simulink model "HPTtest"  (R2025a)
settings: Solver=VariableStepAuto  StartTime=0.0  StopTime=10.0  RelTol=1e-3
undefined symbols (not defined in the file): Eff_hpt_map, effMod_HPT, norm_flow_hpt, norm_speed_hpt, Torque_hpt_map
settings Model: Creator=ramch  LastModifiedBy=ramch

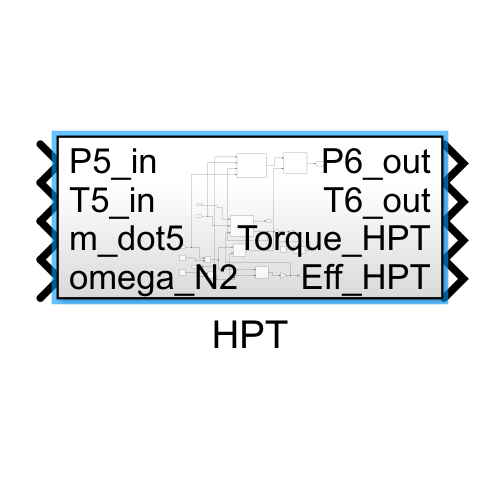
[thumbnail: Simulink's stored preview of the top-level diagram]
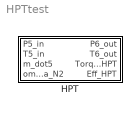
== system HPTtest ==
  HPT : Subsystem

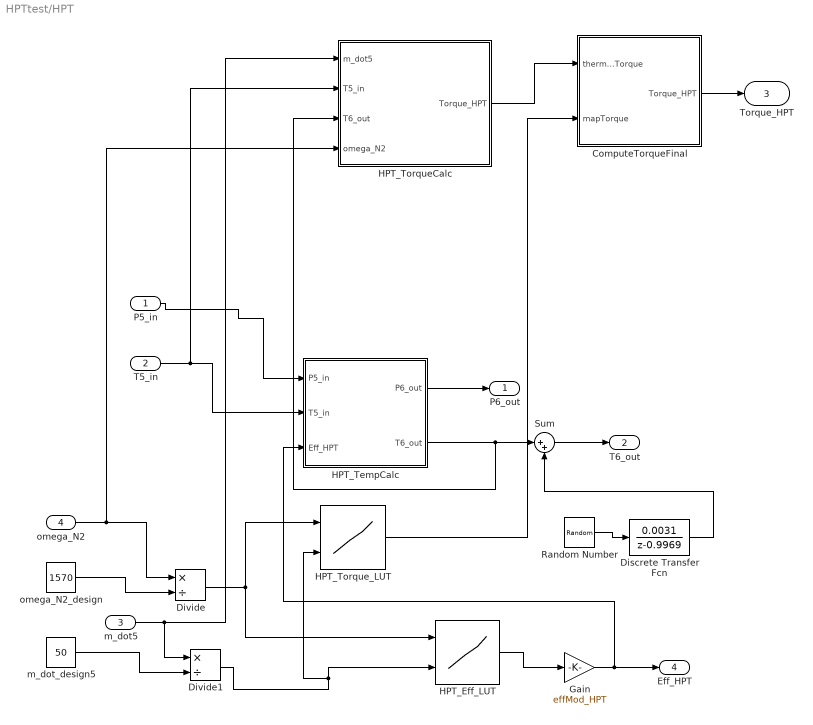
== system HPTtest/HPT ==
  P5_in : Inport
  T5_in : Inport  Port=2
  m_dot5 : Inport  Port=3
  omega_N2 : Inport  Port=4
  ComputeTorqueFinal : MATLAB Function  TreatAsAtomicUnit=on
  Discrete Transfer Fcn : DiscreteTransferFcn  Numerator=0.0031  Denominator=1 -0.9969  InitialStates=0.001
  Divide : Product  Inputs=*/
  Divide1 : Product  Inputs=*/
  Gain : Gain  Gain=effMod_HPT
  HPT_Eff_LUT : Lookup_n-D  BreakpointsForDimension1=norm_speed_hpt  BreakpointsForDimension2=norm_flow_hpt  Table=Eff_hpt_map  InternalRulePriority=Speed  RndMeth=Simplest
      settings: InputPortMap=u0,u1
  HPT_TempCalc : MATLAB Function  TreatAsAtomicUnit=on
  HPT_TorqueCalc : MATLAB Function  TreatAsAtomicUnit=on
  HPT_Torque_LUT : Lookup_n-D  BreakpointsForDimension1=norm_speed_hpt  BreakpointsForDimension2=norm_flow_hpt  Table=Torque_hpt_map  InternalRulePriority=Speed  RndMeth=Simplest
      settings: InputPortMap=u0,u1
  Random Number : RandomNumber  Variance=0.5  SampleTime=0.1
  Sum : Sum  Inputs=|++
  m_dot_design5 : Constant  Value=50
  omega_N2_design : Constant  Value=1570
  P6_out : Outport
  T6_out : Outport  Port=2
  Torque_HPT : Outport  Port=3
  Eff_HPT : Outport  Port=4
  wires:
  m_dot_design5/1 -> Divide1/2
  m_dot5/1 -> HPT_TorqueCalc/1(m_dot5), Divide1/1
  omega_N2_design/1 -> Divide/2
  omega_N2/1 -> HPT_TorqueCalc/4(omega_N2), Divide/1
  Divide/1 -> HPT_Eff_LUT/1, HPT_Torque_LUT/1
  Divide1/1 -> HPT_Torque_LUT/2, HPT_Eff_LUT/2
  P5_in/1 -> HPT_TempCalc/1(P5_in)
  HPT_Eff_LUT/1 -> Gain/1
  Gain/1 -> HPT_TempCalc/3(Eff_HPT), Eff_HPT/1
  T5_in/1 -> HPT_TorqueCalc/2(T5_in), HPT_TempCalc/2(T5_in)
  HPT_TempCalc/1(P6_out) -> P6_out/1
  HPT_TempCalc/2(T6_out) -> HPT_TorqueCalc/3(T6_out), Sum/1
  Discrete Transfer Fcn/1 -> Sum/2
  Sum/1 -> T6_out/1
  Random Number/1 -> Discrete Transfer Fcn/1
  ComputeTorqueFinal/1(Torque_HPT) -> Torque_HPT/1
  HPT_TorqueCalc/1(Torque_HPT) -> ComputeTorqueFinal/1(thermoTorque)
  HPT_Torque_LUT/1 -> ComputeTorqueFinal/2(mapTorque)

== matlab function HPTtest/HPT/HPT_TempCalc ==
  data: P5_in input; P6_out output; T5_in input; Eff_HPT input; T6_out output
function [P6_out, T6_out] = HPT_TempCalc(P5_in, T5_in, Eff_HPT)
    gamma = 1.33;
    PR_turb = 1.0;  % Assume isobaric turbine
    T6_ideal = T5_in * (PR_turb)^((gamma-1)/gamma);
    T6_out = T5_in - Eff_HPT * (T5_in - T6_ideal);
    P6_out = P5_in;  % no pressure drop assumption
end

== matlab function HPTtest/HPT/HPT_TorqueCalc ==
  data: m_dot5 input; Torque_HPT output; T5_in input; T6_out input; omega_N2 input
function Torque_HPT = HPT_TorqueCalc(m_dot5, T5_in, T6_out, omega_N2)
    cp = 1150; % J/kg.K
    work = cp * (T5_in - T6_out); 
    if omega_N2 > 0
        Torque_HPT = (m_dot5 * work) / omega_N2;
    else
        Torque_HPT = 0;
    end
end

== matlab function HPTtest/HPT/ComputeTorqueFinal ==
  data: thermoTorque input; Torque_HPT output; mapTorque input
function Torque_HPT = ComputeTorqueFinal(thermoTorque, mapTorque)
    % Combine both torque calculations with 50/50 weighting
    Torque_HPT = 0.5 * thermoTorque + 0.5 * mapTorque;
end
